simulink library "VsrLibWheel"  (R2019b)
settings: Solver=VariableStepAuto  StartTime=0.0  StopTime=10.0  RelTol=1e-3
settings Model: Creator=9bt  LastModifiedBy=4qz

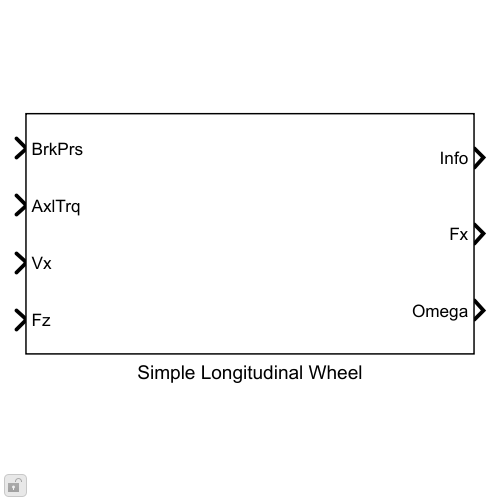
[thumbnail: Simulink's stored preview of the top-level diagram]
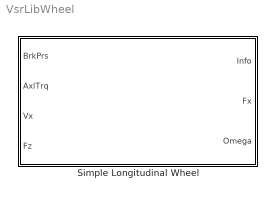
== system VsrLibWheel ==
  Simple Longitudinal Wheel : Subsystem  mask(Simple longitudinal wheel){TireLoadedRadius=0.5, C_rr=.05, MaxBrkTrq=500, MaxBrkPrs=80000, w_thresh=1}
      mask prompts: TireLoadedRadius "Effictive wheel radius, TireLoadedRadius [m]:"; C_rr "Rolling resistance coefficient, C_rr []:"; MaxBrkTrq "Maximum braking torque, MaxBrkTrq [Nm]:"; MaxBrkPrs "Maximum brake pressure, MaxBrkPrs [Pa]:"; w_thresh "Wheel speed threshold for applying brake torque and rolling resistance, w_thresh [rad/s] :"
      mask help: Block implements a simple longitudinal tire and wheel with brakes. Equations assumes no slip and Fz input is only used to calculate the rolling resistance force.

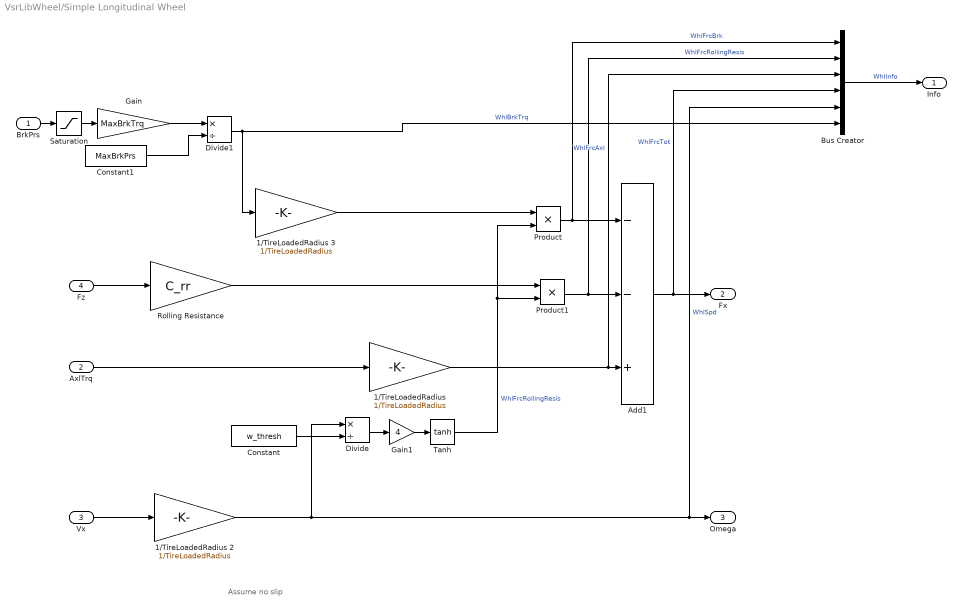
== system VsrLibWheel/Simple Longitudinal Wheel ==
  note: Assume no slip
  BrkPrs : Inport
  AxlTrq : Inport  Port=2
  Vx : Inport  Port=3
  Fz : Inport  Port=4
  1/TireLoadedRadius : Gain  Gain=1/TireLoadedRadius
  1/TireLoadedRadius 2 : Gain  Gain=1/TireLoadedRadius
  1/TireLoadedRadius 3 : Gain  Gain=1/TireLoadedRadius
  Add1 : Sum  Inputs=--+
  Bus Creator : BusCreator  Inputs=6
  Constant : Constant  Value=w_thresh
  Constant1 : Constant  Value=MaxBrkPrs
  Divide : Product  Inputs=*/
  Divide1 : Product  Inputs=*/
  Gain : Gain  Gain=MaxBrkTrq
  Gain1 : Gain  Gain=4
  Product : Product
  Product1 : Product
  Rolling Resistance : Gain  Gain=C_rr
  Saturation : Saturate  UpperLimit=MaxBrkPrs  LowerLimit=0  ZeroCross=off
  Tanh : Trigonometry  Operator=tanh
  Info : Outport
  Fx : Outport  Port=2
  Omega : Outport  Port=3
  wires:
  AxlTrq/1 -> 1/TireLoadedRadius/1
  Fz/1 -> Rolling Resistance/1
  1/TireLoadedRadius 2/1 -> Divide/1, Bus Creator/5, Omega/1  "WhlSpd"
  Vx/1 -> 1/TireLoadedRadius 2/1
  BrkPrs/1 -> Saturation/1
  Constant/1 -> Divide/2
  Divide/1 -> Gain1/1
  Product1/1 -> Bus Creator/2, Add1/2  "WhlFrcRollingResis"
  Add1/1 -> Bus Creator/4, Fx/1  "WhlFrcTot"
  1/TireLoadedRadius/1 -> Bus Creator/3, Add1/3  "WhlFrcAxl"
  Divide1/1 -> 1/TireLoadedRadius 3/1, Bus Creator/6  "WhlBrkTrq"
  1/TireLoadedRadius 3/1 -> Product/1
  Gain1/1 -> Tanh/1
  Product/1 -> Bus Creator/1, Add1/1  "WhlFrcBrk"
  Bus Creator/1 -> Info/1  "WhlInfo"
  Saturation/1 -> Gain/1
  Tanh/1 -> Product/2, Product1/2  "WhlFrcRollingResis"
  Rolling Resistance/1 -> Product1/1
  Gain/1 -> Divide1/1
  Constant1/1 -> Divide1/2
